simulink model "BLDC_V2"  (R2024a)
settings: Solver=ode23tb  StartTime=0.0  StopTime=0.5  MaxStep=1.0E-6  RelTol=1e-3
libraries: spsDCVoltageSourceLib x1, spsPermanentMagnetSynchronousMachineLib x1, spsUniversalBridgeLib x1, sps_lib x1
settings Model: Creator=18283  LastModifiedBy=18283

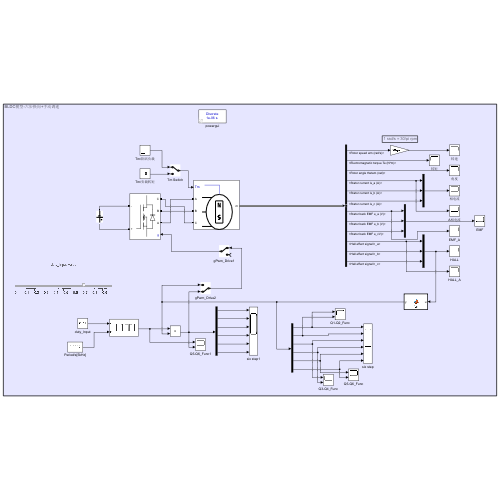
[thumbnail: Simulink's stored preview of the top-level diagram]
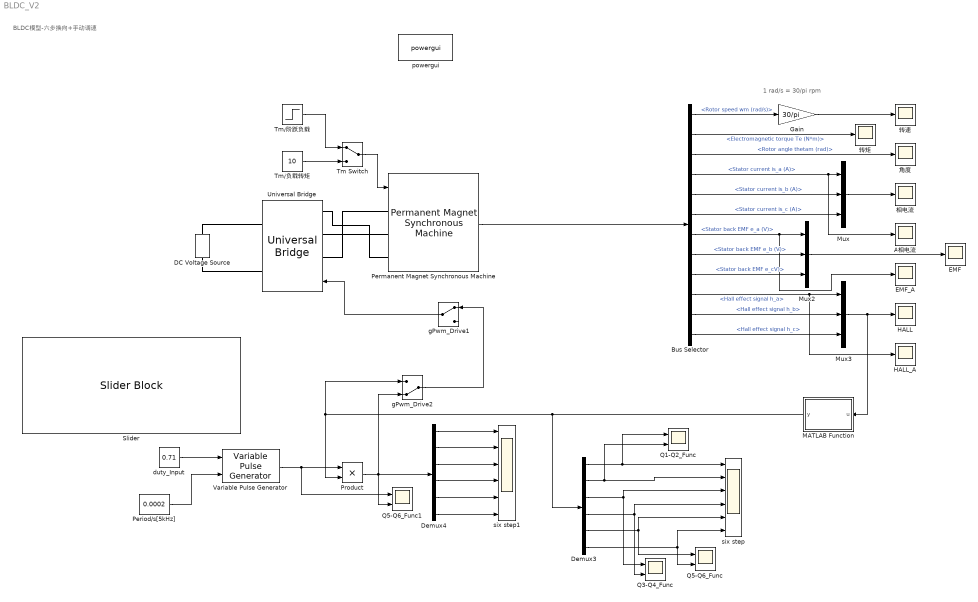
== system BLDC_V2 ==
  note: BLDC模型-六步换向+手动调速
  note: 1 rad/s = 30/pi rpm
  A相电流 : Scope
  Bus Selector : BusSelector  OutputSignals=Rotor speed wm (rad/s),Electromagnetic torque Te (N*m),Rotor angle thetam (rad),Stator current is_a (A),Stator current is_b (A),Stator current is_c (A),Stator back EMF e_a (V),Stator back EMF e_b (V),Stator back EMF e_cV),Hall effect signal h_a,Hall effect signal h_b,Hall effect signal h_c
  DC Voltage Source : spsDCVoltageSourceLib/DC Voltage Source  Amplitude=560  Measurements=None
  Demux3 : Demux  Outputs=6
  Demux4 : Demux  Outputs=6
  EMF : Scope
  EMF_A : Scope
  Gain : Gain  Gain=30/pi
  HALL : Scope
  HALL_A : Scope
  MATLAB Function : MATLAB Function  TreatAsAtomicUnit=on
  Mux : Mux  Inputs=3
  Mux2 : Mux  Inputs=3
  Mux3 : Mux  Inputs=3
  Period/s[5kHz] : Constant  Value=0.0002
  Permanent Magnet Synchronous Machine : spsPermanentMagnetSynchronousMachineLib/Permanent Magnet Synchronous Machine  NbPhases=3  FluxDistribution=Trapezoidal  RotorType=Round  MechanicalLoad=Torque Tm  PresetModel="11:  26.13 Nm 560 Vdc 3000 RPM - 27.3 Nm"  ShowDetailedParameters=on  MeasurementBus=off  Resistance=0.11  Inductance=8.5e-3  dqInductances=[8.5e-3,8.5e-3]  La=0.00097  MachineConstant=Flux linkage established by magnets (V.s)  Flux=0.1119  VoltageCst=93.7451  TorqueCst=0.8952  Flat=120  Mechanical=[0.0016 0.0002024 4 0.5]  PolePairs=4  InitialConditions=[0,0, 0,0]  InitialConditions5ph=[0 0 0 0 0 0]  RefAngle=Aligned with phase A axis (original Park)  IterativeDiscreteModel=Trapezoidal non iterative  TsBlock=-1  TsPowergui=0
  Product : Product
  Q1-Q2_Func : Scope  NumInputPorts=2
  Q3-Q4_Func : Scope  NumInputPorts=2
  Q5-Q6_Func : Scope  NumInputPorts=2
  Q5-Q6_Func1 : Scope  NumInputPorts=2
  Slider : SliderBlock  ScaleMax=1
  Tm Switch : ManualSwitch
  Tm/负载转矩 : Constant  Value=10
  Tm/阶跃负载 : Step  Time=0.25  After=10  SampleTime=0
  Universal Bridge : spsUniversalBridgeLib/Universal Bridge  Arms=3  SnubberResistance=1e5  SnubberCapacitance=inf  Device=MOSFET / Diodes  Ron=1e-3  Lon=0  ForwardVoltages="[  0  0  ]"  ForwardVoltage=0  GTOparameters=[ 10e-6 , 20e-6 ]  IGBTparameters=[ 1e-6 , 2e-6 ]  Measurements=None  Measurements_2=None  converterType=Rectifier
  Variable Pulse Generator : VariablePulseGenerator  SampleTime=0.1
  duty_Input : Constant  Value=0.71
  gPwm_Drive1 : ManualSwitch
  gPwm_Drive2 : ManualSwitch  CurrentSetting=0
  powergui : sps_lib/powergui  Priority=1  SimulationMode=Discrete  SampleTime=1e-6  frequency=60  Iterations=50  frequencyindice=0  Pbase=100e6  ErrMax=1e-4  UnitsV=kV  UnitsW=MW  buscounter=0  FunctionMessages=off  echomessages=off  EnableUseOfTLC=off  CurrentSourceSwitches=off  DisableSnubberDevices=off  DisableRonSwitches=off  DisableVfSwitches=off  DisplayEquations=off  AutomaticDiscreteSolvers=off  SolverType=Tustin/Backward Euler (TBE)  Interpol=off  ExternalGateDelay=off  methode=off  Ts=100  x0status=blocks  SPID=on  SwTol=0  HookPort=off  NonlinearTolerance=1e-4  nMaxIteration=100  ContinueOnMaxIteration=off  RestoreLinks=warning  ResistiveCurrentMeasurement=off  Frange=[0:2:500]  Ylog=off  Xlog=on  ShowGrid=off  save=off  variable=ZData  structure=0  ZoomFFT=off  StartTime=0.0  cycles=1  DisplayStyle=1  fundamental=60  FreqAxis=off  MaxFrequency=1000  frequencyindicesteady=1  RmsSteady=1  display=off
  six step : Scope  NumInputPorts=6
  six step1 : Scope  NumInputPorts=6
  相电流 : Scope
  角度 : Scope
  转矩 : Scope
  转速 : Scope
  wires:
  gPwm_Drive1/1 -> Universal Bridge/1
  gPwm_Drive2/1 -> gPwm_Drive1/1
  Tm Switch/1 -> Permanent Magnet Synchronous Machine/1
  Tm/阶跃负载/1 -> Tm Switch/1
  Demux4/3 -> six step1/3
  Demux4/1 -> six step1/1
  Demux4/6 -> six step1/6
  Demux4/4 -> six step1/4
  Demux3/2 -> Q1-Q2_Func/2, six step/2
  Product/1 -> gPwm_Drive2/2, Q5-Q6_Func1/2, Demux4/1
  Demux4/5 -> six step1/5
  Period/s[5kHz]/1 -> Variable Pulse Generator/2
  duty_Input/1 -> Variable Pulse Generator/1
  Demux3/4 -> six step/4, Q3-Q4_Func/2
  Bus Selector/4 -> A相电流/1, Mux/1  "<Stator current is_a (A)>"
  Demux3/1 -> Q1-Q2_Func/1, six step/1
  Mux/1 -> 相电流/1
  Tm/负载转矩/1 -> Tm Switch/2
  Bus Selector/1 -> Gain/1  "<Rotor speed wm (rad/s)>"
  Variable Pulse Generator/1 -> Q5-Q6_Func1/1, Product/1
  Bus Selector/8 -> Mux2/2  "<Stator back EMF e_b (V)>"
  Demux3/5 -> Q5-Q6_Func/1, six step/5
  Demux3/3 -> Q3-Q4_Func/1, six step/3
  Bus Selector/2 -> 转矩/1  "<Electromagnetic torque Te (N*m)>"
  MATLAB Function/1(y) -> Demux3/1, Product/2, gPwm_Drive2/1
  Gain/1 -> 转速/1
  Mux2/1 -> EMF/1
  Mux3/1 -> MATLAB Function/1(u), HALL/1
  Permanent Magnet Synchronous Machine/1 -> Bus Selector/1
  Bus Selector/10 -> HALL_A/1, Mux3/1  "<Hall effect signal h_a>"
  Bus Selector/5 -> Mux/2  "<Stator current is_b (A)>"
  Bus Selector/11 -> Mux3/2  "<Hall effect signal h_b>"
  Bus Selector/7 -> EMF_A/1, Mux2/1  "<Stator back EMF e_a (V)>"
  Bus Selector/12 -> Mux3/3  "<Hall effect signal h_c>"
  Bus Selector/6 -> Mux/3  "<Stator current is_c (A)>"
  Demux3/6 -> six step/6, Q5-Q6_Func/2
  Bus Selector/9 -> Mux2/3  "<Stator back EMF e_cV)>"
  Bus Selector/3 -> 角度/1  "<Rotor angle thetam (rad)>"
  Demux4/2 -> six step1/2
  connections:
  DC Voltage Source/LConn1 -- Universal Bridge/RConn2
  Universal Bridge/LConn3 -- Permanent Magnet Synchronous Machine/LConn3
  Universal Bridge/LConn1 -- Permanent Magnet Synchronous Machine/LConn1
  Universal Bridge/LConn2 -- Permanent Magnet Synchronous Machine/LConn2
  DC Voltage Source/RConn1 -- Universal Bridge/RConn1

== matlab function BLDC_V2/MATLAB Function ==
  data: u input; y output
function y = fcn(u)
    index = u(1)*4 + u(2)*2 + u(3);
    switch index
        case 1%'001'  % 状态 001 → Q4, Q5 导通
            y = [0, 0, 0, 1, 1, 0];
        case 2%'010'  % 状态 010 → Q2, Q3 导通
            y = [0, 1, 1, 0, 0, 0];
        case 3%'011'  % 状态 011 → Q3, Q4 导通
            y = [0, 1, 0, 0, 1, 0];
        case 4%'100'  % 状态 100 → Q5, Q4 导通
            y = [1, 0, 0, 0, 0, 1];
        case 5%'101'  % 状态 101 → Q5, Q2 导通
            y = [1, 0, 0, 1, 0, 0];
        case 6%'110'  % 状态 110 → Q1, Q2 导通
            y = [0, 0, 1, 0, 0, 1];
        otherwise   % 无效状态（如 000, 111）→ 全关断
            y = [0, 0, 0, 0, 0, 0];
    end
end
